simulink model "Sym_ex_4"  (R2021b)
settings: Solver=VariableStepAuto  StartTime=0.0  StopTime=30  RelTol=1e-3
values from neighbouring files (symbols this model uses):
  k = 2    [Ex_4.m]
settings Model: Creator=Leonardo  LastModifiedBy=Leonardo
settings DataIOCC: Refine=1000

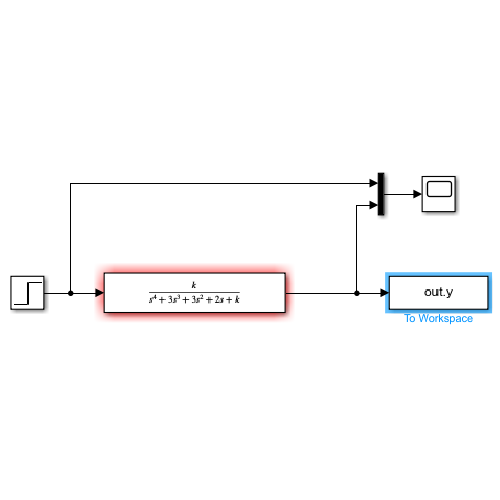
[thumbnail: Simulink's stored preview of the top-level diagram]
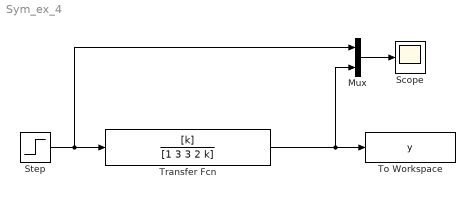
== system Sym_ex_4 ==
  Mux : Mux  Inputs=2
  Scope : Scope
  Step : Step  Time=0  SampleTime=0
  To Workspace : ToWorkspace  VariableName=y  SaveFormat=Structure With Time  SampleTime=-1
  Transfer Fcn : TransferFcn  Numerator=[k]  Denominator=[1 3 3 2 k]
  wires:
  Mux/1 -> Scope/1
  Transfer Fcn/1 -> To Workspace/1, Mux/2
  Step/1 -> Mux/1, Transfer Fcn/1
